simulink model "blocks"  (R2019a)
settings: Solver=VariableStepAuto  StartTime=0.0  StopTime=10.0  RelTol=1e-3
settings Model: Creator=adeye  LastModifiedBy=adeye

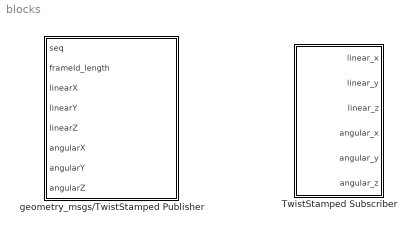
== system blocks ==
  TwistStamped Subscriber : Subsystem  mask{topic='/TwistS', message_type='geometry_msgs/TwistStamped', port=9090, timeout=2}
      mask prompts: topic "Topic name"; message_type "Message type"; timeout "Timeout (s)"
  geometry_msgs/TwistStamped Publisher : Subsystem  mask{topic='/current_velocity', message_type='geometry_msgs/TwistStamped', port=9090, timeout=2}
      mask prompts: topic "Topic name"; message_type "Message type"; timeout "Timeout (s)"

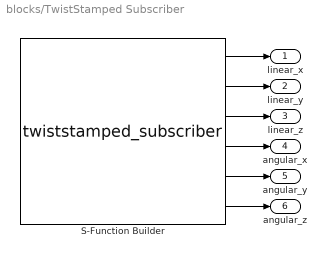
== system blocks/TwistStamped Subscriber ==
  S-Function Builder : S-Function  InitFcn=try, set_param(gcb,'FunctionName','twiststamped_subscriber'), end  FunctionName=twiststamped_subscriber  Parameters=int8(topic),int8(message_type),port,timeout  SFunctionModules=twiststamped_subscriber_wrapper rosbridge_functions  SFunctionDeploymentMode=off  EnableBusSupport=off  mask(S-Function Builder){}
      mask help: Simulink:masks:SFunctionBuilder_MD
      mask init:
      | val = [[.9  0.75 0.75 1 1 .9 .9 1]',[1 1 0.75 0.75 .9 .9 1 .9]'];try , sys = get_param(gcb,'SfunBuilderFcnName');if isempty(sys), sys = get_param(gcb,'FunctionName'); end,catch, sys = get_param(gcb,'FunctionName'); end
      settings: CopyFcn=set_param(gcbh,'LinkStatus','none')  PreSaveFcn=try, set_param(gcb,'FunctionName','twiststamped_subscriber'), end  OpenFcn=sfunctionwizard(gcbh)
      mask Display: plot(val(:,1),val(:,2)),disp(sys), port_label('output',1,'linear_x'), port_label('output',2,'linear_y'), port_label('output',3,'linear_z'), port_label('output',4,'angular_x'), port_label('output',5,'angular_y'), port_label('output',6,'angular_z')
  linear_x : Outport
  linear_y : Outport  Port=2
  linear_z : Outport  Port=3
  angular_x : Outport  Port=4
  angular_y : Outport  Port=5
  angular_z : Outport  Port=6
  wires:
  S-Function Builder/1 -> linear_x/1
  S-Function Builder/2 -> linear_y/1
  S-Function Builder/3 -> linear_z/1
  S-Function Builder/4 -> angular_x/1
  S-Function Builder/5 -> angular_y/1
  S-Function Builder/6 -> angular_z/1

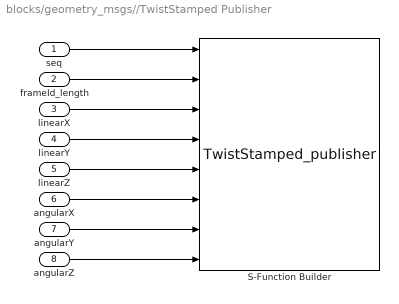
== system blocks/geometry_msgs//TwistStamped Publisher ==
  seq : Inport
  frameId_length : Inport  Port=2
  linearX : Inport  Port=3
  linearY : Inport  Port=4
  linearZ : Inport  Port=5
  angularX : Inport  Port=6
  angularY : Inport  Port=7
  angularZ : Inport  Port=8
  S-Function Builder : S-Function  InitFcn=try, set_param(gcb,'FunctionName','TwistStamped_publisher'), end  FunctionName=TwistStamped_publisher  Parameters=int8(topic),int8(message_type),port,timeout  SFunctionModules=TwistStamped_publisher_wrapper rosbridge_functions  SFunctionDeploymentMode=off  EnableBusSupport=off  mask(S-Function Builder){}
      mask help: Simulink:masks:SFunctionBuilder_MD
      mask init: same as blocks/TwistStamped Subscriber/S-Function Builder
      settings: CopyFcn=set_param(gcbh,'LinkStatus','none')  PreSaveFcn=try, set_param(gcb,'FunctionName','TwistStamped_publisher'), end  OpenFcn=sfunctionwizard(gcbh)
      mask Display: plot(val(:,1),val(:,2)),disp(sys), port_label('input',1,'seq'), port_label('input',2,'frameId_length'), port_label('input',3,'linearX'), port_label('input',4,'linearY'), port_label('input',5,'linearZ'), port_label('input',6,'angularX'), port_label('input',7,'angularY'), port_label('input',8,'angularZ')
  wires:
  seq/1 -> S-Function Builder/1
  frameId_length/1 -> S-Function Builder/2
  linearX/1 -> S-Function Builder/3
  linearY/1 -> S-Function Builder/4
  linearZ/1 -> S-Function Builder/5
  angularX/1 -> S-Function Builder/6
  angularY/1 -> S-Function Builder/7
  angularZ/1 -> S-Function Builder/8
